simulink model "untitled1"  (R2018a)
settings: Solver=VariableStepAuto  StartTime=0.0  StopTime=600  FixedStep=0.001  MinStep=0.001  RelTol=1e-3
settings Model: Creator=kyniu  LastModifiedBy=kyniu
settings DataIOCC: LimitDataPoints=on  MaxDataPoints=3  SaveOutput=off  SignalLogging=off  DSMLogging=off
settings DebuggingCC: AlgebraicLoopMsg=none  ArtificialAlgebraicLoopMsg=none  MaxConsecutiveZCsMsg=none  ModelReferenceExtraNoncontSigs=none  SimStateInterfaceChecksumMismatchMsg=none
settings RTWCC: Toolchain=Microsoft Visual C++ 2015 v14.0 | nmake (64-bit Windows)  BuildConfiguration=Faster Runs  CheckMdlBeforeBuild=Warning

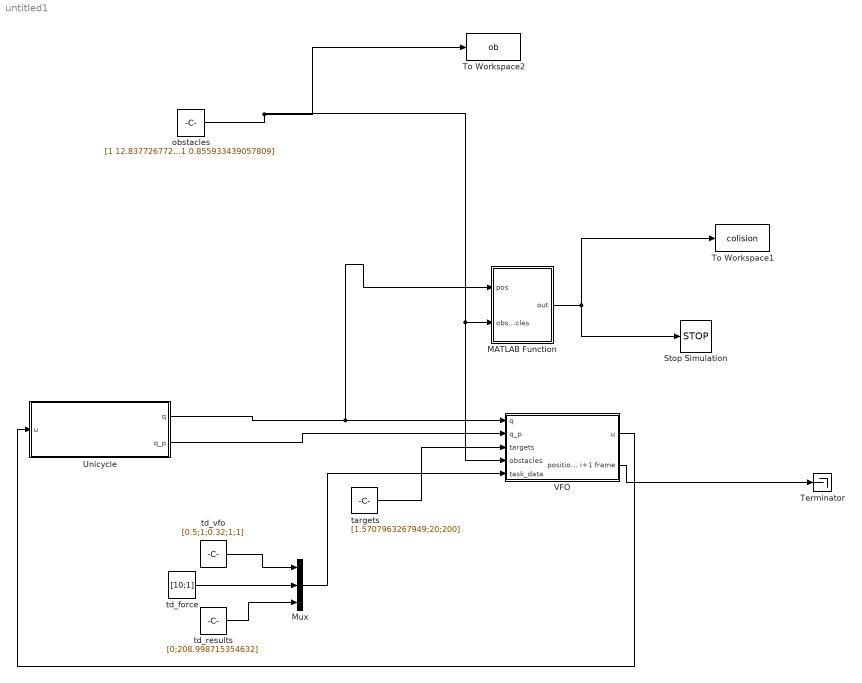
== system untitled1 ==
  MATLAB Function : MATLAB Function  TreatAsAtomicUnit=on
  Mux : Mux  Inputs=3
  Stop Simulation : Stop
  Terminator : Terminator
  To Workspace1 : ToWorkspace  VariableName=colision  SaveFormat=Timeseries  SampleTime=-1
      settings: MaxDataPoints=3
  To Workspace2 : ToWorkspace  VariableName=ob  SaveFormat=Timeseries  SampleTime=-1
  Unicycle : Subsystem
  VFO : Subsystem
  obstacles : Constant  Value=[1 12.8377267725443 84.352256525255 4.57867762594534;2 25.8441465911911 191.898485278581 3.27870349578293;3 10.7142335714838 169.825861173755 4.66996623878775;4 23.5747030971555 151.548026115667 3.71566234062458;5 17.8445403906834 131.095578035511 0.855933439057809]  VectorParams1D=off
  targets : Constant  Value=[1.5707963267949;20;200]
  td_force : Constant  Value=[10;1]
  td_results : Constant  Value=[0;208.998715354632]
  td_vfo : Constant  Value=[0.5;1;0.32;1;1]
  wires:
  VFO/1("u ") -> Unicycle/1(u)
  Unicycle/2(q_p) -> VFO/2(q_p)
  Unicycle/1(q) -> VFO/1(q), MATLAB Function/1(pos)
  MATLAB Function/1(out) -> Stop Simulation/1, To Workspace1/1
  VFO/2(position in i+1 frame) -> Terminator/1
  obstacles/1 -> VFO/4(obstacles), MATLAB Function/2(obstacles), To Workspace2/1
  targets/1 -> VFO/3(targets)
  td_vfo/1 -> Mux/1
  td_force/1 -> Mux/2
  td_results/1 -> Mux/3
  Mux/1 -> VFO/5("task_data ")

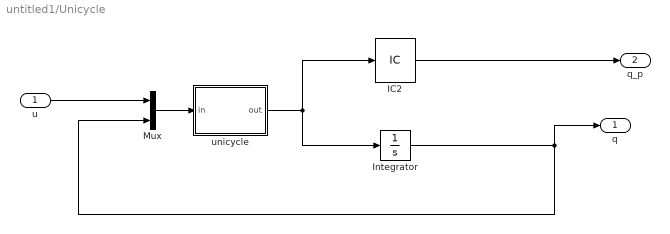
== system untitled1/Unicycle ==
  u : Inport
  IC2 : InitialCondition  Value=[0;0;0]
  Integrator : Integrator  InitialCondition=[pi/2, 20, 0]
  Mux : Mux  Inputs=2
  unicycle : MATLAB Function  TreatAsAtomicUnit=on
  q : Outport
  q_p : Outport  Port=2
  wires:
  Integrator/1 -> q/1, Mux/2
  IC2/1 -> q_p/1
  Mux/1 -> unicycle/1(in)
  unicycle/1(out) -> Integrator/1, IC2/1
  u/1 -> Mux/1

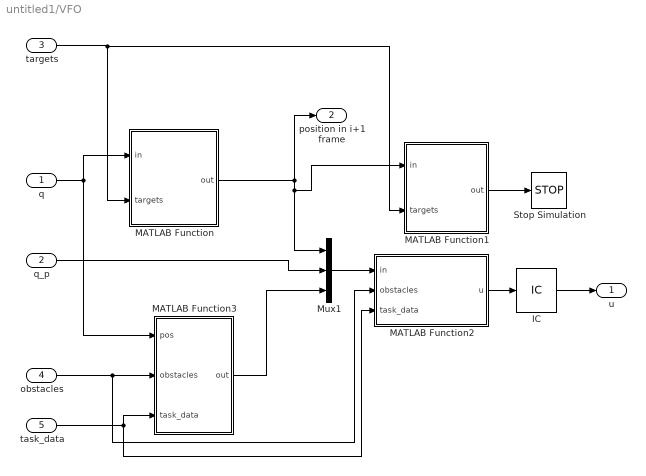
== system untitled1/VFO ==
  q : Inport  PortDimensions=3
  q_p : Inport  Port=2
  targets : Inport  Port=3
  obstacles : Inport  Port=4
  "task_data " : Inport  Port=5
  IC : InitialCondition  Value=[0;0]
  MATLAB Function : MATLAB Function  TreatAsAtomicUnit=on
  MATLAB Function1 : MATLAB Function  TreatAsAtomicUnit=on
  MATLAB Function2 : MATLAB Function  TreatAsAtomicUnit=on
  MATLAB Function3 : MATLAB Function  TreatAsAtomicUnit=on
  Mux1 : Mux  Inputs=3
  Stop Simulation : Stop
  "u " : Outport
  position in i+1 frame : Outport  Port=2
  wires:
  Mux1/1 -> MATLAB Function2/1(in)
  MATLAB Function2/1(u) -> IC/1
  IC/1 -> "u "/1
  q_p/1 -> Mux1/2
  MATLAB Function/1(out) -> position in i+1 frame/1, MATLAB Function1/1(in), Mux1/1
  q/1 -> MATLAB Function3/1(pos), MATLAB Function/1(in)
  MATLAB Function3/1(out) -> Mux1/3
  MATLAB Function1/1(out) -> Stop Simulation/1
  targets/1 -> MATLAB Function1/2(targets), MATLAB Function/2(targets)
  obstacles/1 -> MATLAB Function3/2(obstacles), MATLAB Function2/2(obstacles)
  "task_data "/1 -> MATLAB Function2/3(task_data), MATLAB Function3/3(task_data)

== matlab function untitled1/MATLAB Function ==
  data: pos input; out output; obstacles input
function out  = isColision(pos, obstacles)
%ISCOLISION Summary of this function goes here
%   Detailed explanation goes here
%global obstacles

out = 0;
for i = 1:size(obstacles,1)
        obstacle = obstacles(i, :);
    dist = sqrt((pos(2)-obstacle(2))^2 + (pos(3)-obstacle(3))^2);
    if dist < obstacle(4)
        out = 1;
    end
end

== matlab function untitled1/Unicycle/unicycle ==
  data: in input; out output
function out  = unicycle(in)
%kinematics of aan unicycle

u = in(1:2);
q = in(3:5);

q_p = [1;0;0]*u(1)+[0;cos(q(1));sin(q(1))]*u(2);
out = q_p; 
end

== matlab function untitled1/VFO/MATLAB Function ==
  data: in input; out output; targets input
function out  = globtonextframe(in, targets)
%GLOBTONEXTFRAME Summary of this function goes here
%   Detailed explanation goes here
%global targets targetIter
targetIter = 1;
q_glob = in(1:3);
i_glob = targets(:,targetIter);

R = [cos(i_glob(1)), -sin(i_glob(1));...
    sin(i_glob(1)), cos(i_glob(1))];

pos_new = R\(q_glob(2:3)-i_glob(2:3));
th_new = q_glob(1)-i_glob(1);
out = [th_new; pos_new];


end

== matlab function untitled1/VFO/MATLAB Function1 ==
  data: in input; out output; targets input
function out  = isNearEnd(in, targets)
%ISNEAREND Summary of this function goes here
%   Detailed explanation goes here
pos = in(1:3);
%global targets targetIter
targetIter = 1;
out = 0;
if norm(pos(2:3)) < 1
%     targetIter = targetIter+1;
%     if targetIter > size(targets, 2)
%         targetIter = size(targets, 2);
%     end
    out = 1;
end
% target = targets(:,targetIter);
% out = target;
end

== matlab function untitled1/VFO/MATLAB Function2 ==
  data: in input; u output; obstacles input; task_data input
function u  = VFO(in, obstacles, task_data)
%global obstacles task_data
%VFO Summary of this function goes here
%   Detailed explanation goes here

qi = in(1:3);
q_p = in(4:6);
forceField = in(7);

qi_p = q_p;%globtonextframe(q_p, target)
%qi_p(1) = th_p

vfo_kp = task_data(1);
vfo_ka = task_data(2);
vfo_eta = task_data(3);
%mii = 0.65;
vfo_sigmai = task_data(4);
vfo_U2 = task_data(5);
%kb = 0.6;



roi = vfo_U2;
mii = vfo_eta*vfo_kp^(-1);
vdi = -vfo_kp*mii*vfo_sigmai*norm(qi(2:3))*[1;0];
hdi = -vfo_kp*qi(2:3)+vdi;
thai = atan2(vfo_sigmai * hdi(2), vfo_sigmai*hdi(1));
eai = thai - qi(1);  

%%needed for thai_p only
v_p = -vfo_kp*mii*vfo_sigmai*((qi(2:3)'*(qi_p(2:3))))/norm((qi(2:3)))*[1;0];
hdi_p = -vfo_kp*(qi_p(2:3))+v_p;
thai_p = (hdi_p(2)*hdi(1)-hdi_p(1)*hdi(2))/(hdi(1)^2+hdi(2)^2);


hai = vfo_ka*eai + thai_p + forceField;%q_p(1);
if norm(qi(2:3)) > 0.5
    u = [hai; roi*vfo_sigmai*cos(eai)];
else
    u = [0;0];
end

end

== matlab function untitled1/VFO/MATLAB Function3 ==
  data: pos input; out output; obstacles input; task_data input
function out  = calcForceField(pos, obstacles, task_data)
%UNTITLED Summary of this function goes here
%   Detailed explanation goes here
%global obstacles task_data
k = 1;
%%task_function = '1*sign/dist'
activationDistance = task_data(6);
force = 0;
for i = 1:size(obstacles,1)
    dist = getDistFromObstacle(obstacles(i,:), pos);
    sign = getObstacleSide(obstacles(i,:), pos);
    if dist < activationDistance
        force = force + 1*sign/dist; %eval(task_function);
        %force = force + sign*1/dist;
        %force = force + sign*(activationDistance-dist);
    end
end
%account for left border
dist = getDistFromObstacle([0, 10, pos(3), 0], pos);
sign = getObstacleSide([0, 10, pos(3), 0], pos);
force = force + 1*sign/dist; % eval(task_function);
%account for right border
dist = getDistFromObstacle([0, 30, pos(3), 0], pos);
sign = getObstacleSide([0, 30, pos(3), 0], pos);
force = force + 1*sign/dist; %eval(task_function);
out = force;
end
